simulink model "rocket"  (R2021a)
settings: Solver=VariableStepAuto  StartTime=0.0  StopTime=40  RelTol=1e-3
libraries: dspindex x5, shared3dof x3, aerolibanim x2
settings Model: Creator=scien  LastModifiedBy=scien
settings SolverCC: ZeroCrossAlgorithm=Adaptive
settings DebuggingCC: IgnoredZcDiagnostic=none

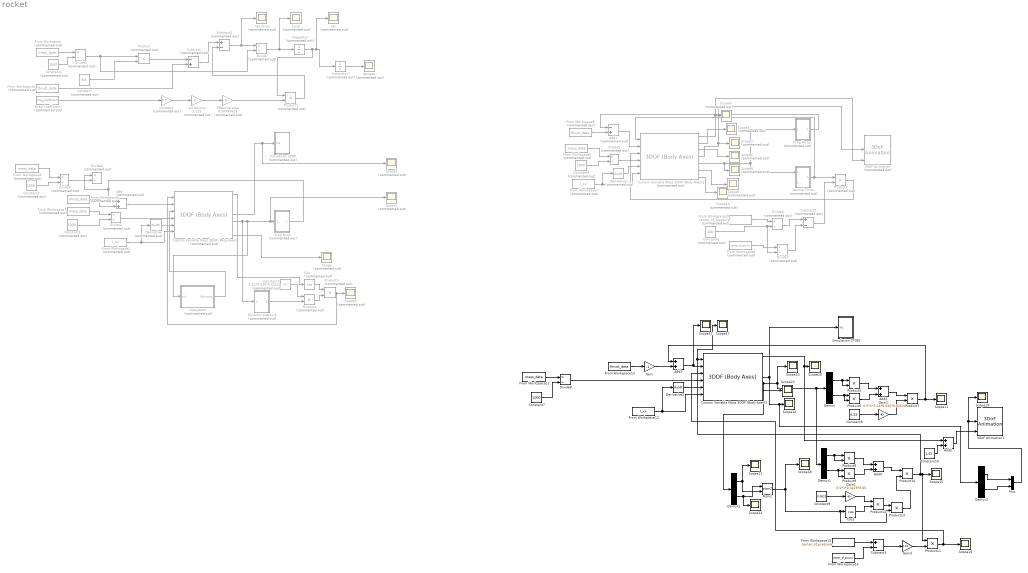
== system rocket ==
  3DoF Animation : aerolibanim/3DoF Animation  Commented=on  u1=[0 5000 -2000 2000 -5050 -3050]  u2=0.05  u3=1.0  u5=Fixed position  u6=[2000 500 -3150]  u7=10  u8=on
      settings: SourceProductBaseCode=AE
  3DoF Animation1 : aerolibanim/3DoF Animation  u1=[0 5000 -2000 2000 -5050 -3050]  u2=0.005  u3=1.0  u5=Fly alongside  u6=[0 2000 0]  u7=10  u8=on
      settings: SourceProductBaseCode=AE
  Add : Sum  Commented=on
  Add1 : Sum  Commented=on  Inputs=-+
  Add{2..5} (4 alike) : Sum
  Apogee : Scope  Commented=on
  Atan2 : Trigonometry  Operator=atan2  OutputSignalType=real
  Constant : Constant  Commented=on  Value=9.8
  Constant{1..2,4..5} (4 alike) : Constant  Commented=on  Value=1000
  Constant10 : Constant  Value=1.57
  Constant3 : Constant  Commented=on  Value=3.14*0.025*0.025/4
  Constant6 : Constant  Commented=on  Value=100
  Constant7 : Constant  Value=1000
  Constant8 : Constant  Value=6.25
  Constant9 : Constant  Value=0.0625
  Cos : Trigonometry  Commented=on  Operator=cos
  Cos1 : Trigonometry  Operator=cos
  Custom Variable Mass 3DOF (Body Axes) : shared3dof/3DOF (Body Axes)  Commented=on  units=Metric (MKS)  mtype=Custom Variable  v_ini=0  theta_ini=0  alpha_ini=0  pos_ini=[0 0]  q_ini=0  mass=1.0  mass_e=0.5  mass_f=3.0  Iyy=1.0  Iyy_e=0.5  Iyy_f=3.0  g_in=Internal  g=-9.81  vre_flag=off  abi_flag=on  aMode=0  vel_statename=''  theta_statename=''  pos_statename=''  q_statename=''  mass_statename=''
      settings: SourceProductBaseCode=AE,PW,DR,MT,UV,VE
  Custom Variable Mass 3DOF (Body Axes)1 : shared3dof/3DOF (Body Axes)  Commented=on  units=Metric (MKS)  mtype=Custom Variable  v_ini=0  theta_ini=0  alpha_ini=0  pos_ini=[0 0]  q_ini=0  mass=1.0  mass_e=0.5  mass_f=3.0  Iyy=1.0  Iyy_e=0.5  Iyy_f=3.0  g_in=Internal  g=-9.81  vre_flag=off  abi_flag=on  aMode=0  vel_statename=''  theta_statename=''  pos_statename=''  q_statename=''  mass_statename=''
      settings: SourceProductBaseCode=AE,PW,DR,MT,UV,VE
  Custom Variable Mass 3DOF (Body Axes)2 : shared3dof/3DOF (Body Axes)  units=Metric (MKS)  mtype=Custom Variable  v_ini=0  theta_ini=-0.2  alpha_ini=0  pos_ini=[0 0]  q_ini=0  mass=1.0  mass_e=0.5  mass_f=3.0  Iyy=1.0  Iyy_e=0.5  Iyy_f=3.0  g_in=Internal  g=9.81  vre_flag=off  abi_flag=on  aMode=0  vel_statename=''  theta_statename=''  pos_statename=''  q_statename=''  mass_statename=''
      settings: SourceProductBaseCode=AE,PW,DR,MT,UV,VE
  Demux{,1..3} (4 alike) : Demux  Outputs=2
  Derivative : Derivative  Commented=on
  Derivative1 : Derivative  Commented=on
  Derivative2 : Derivative
  Divide{,1..7} (8 alike) : Product  Commented=on  Inputs=*/
  Divide8 : Product  Inputs=*/
  Drag Coefficient : FromWorkspace  Commented=on  VariableName=drag_coefficient
  Drag Force : Subsystem  Commented=on
  Dynamic pressure : Subsystem  Commented=on
  Effective area : Gain  Commented=on  Gain=0.00490625
  From Workspace{,3,5..6} (4 alike) : FromWorkspace  Commented=on  VariableName=mass_data
  From Workspace1 : FromWorkspace  Commented=on  VariableName=thrust_data
  From Workspace10 : FromWorkspace  Commented=on  VariableName=center_of_pressure
  From Workspace11 : FromWorkspace  VariableName=mass_data
  From Workspace12 : FromWorkspace  VariableName=I_xx
  From Workspace13 : FromWorkspace  VariableName=thrust_data
  From Workspace14 : FromWorkspace  VariableName=center_of_gravity
  From Workspace15 : FromWorkspace  VariableName=center_of_pressure
  From Workspace2 : FromWorkspace  Commented=on  VariableName=I_xx
  From Workspace4 : FromWorkspace  Commented=on  VariableName=thrust_data
  From Workspace7 : FromWorkspace  Commented=on  VariableName=I_xx
  From Workspace8 : FromWorkspace  Commented=on  VariableName=thrust_data
  From Workspace9 : FromWorkspace  Commented=on  VariableName=center_of_gravity
  Gain : Gain  Gain=-1
  Gain1 : Gain  Gain=0.5*1*3.14*0.025*0.025/4
  Gain2 : Gain  Gain=0.5*1*0.3225*0.05
  Gain3 : Gain  Gain=0.01
  Integrator : Integrator  Commented=on
  Integrator1 : Integrator  Commented=on
  Mux : Mux  Inputs=2
  Normal Force : Subsystem  Commented=on
  Product{,1..4} (5 alike) : Product  Commented=on
  Product{5..13} (9 alike) : Product
  Scope{,1..10} (11 alike) : Scope  Commented=on
  Scope{11..23} (13 alike) : Scope
  Simulation STOP : Subsystem  Commented=on
  Simulation STOP2 : Subsystem
  Subsystem : Subsystem  Commented=on
  Subtract : Sum  Commented=on  Inputs=-+
  Subtract1 : Sum  Commented=on  Inputs=+-
  Subtract2 : Sum  Commented=on  Inputs=+-
  Subtract3 : Sum  Inputs=+-
  accel : Scope  Commented=on
  air density : Gain  Commented=on  Gain=1.225
  constant : Gain  Commented=on  Gain=0.5
  drag force : Subsystem  Commented=on
  net_force : Scope  Commented=on
  vel : Scope  Commented=on
  wires:
  Constant/1 -> Product/2
  From Workspace1/1 -> Subtract/2
  Product/1 -> Subtract/1
  Divide/1 -> accel/1, Integrator/1
  Integrator/1 -> vel/1, Integrator1/1, Product1/1
  Integrator1/1 -> Apogee/1
  Constant1/1 -> Divide1/2
  Divide1/1 -> Divide/2, Product/1
  From Workspace/1 -> Divide1/1
  Drag Coefficient/1 -> constant/1
  constant/1 -> air density/1
  air density/1 -> Effective area/1
  Effective area/1 -> Product1/2
  Subtract/1 -> Subtract1/1
  Product1/1 -> Subtract1/2
  Subtract1/1 -> net_force/1, Divide/1
  From Workspace2/1 -> Derivative/1, Custom Variable Mass 3DOF (Body Axes)/6
  Derivative/1 -> Custom Variable Mass 3DOF (Body Axes)/5
  From Workspace3/1 -> Divide2/1
  Constant4/1 -> Divide2/2
  Divide2/1 -> Custom Variable Mass 3DOF (Body Axes)/4
  From Workspace4/1 -> Add/2
  Add/1 -> Custom Variable Mass 3DOF (Body Axes)/2
  Custom Variable Mass 3DOF (Body Axes)/4 -> Simulation STOP/1(In1), Scope2/1
  drag force/1(Out2) -> Divide4/1, Add/1
  Subsystem/1(Moments) -> Custom Variable Mass 3DOF (Body Axes)/3
  From Workspace5/1 -> Divide3/1
  Constant2/1 -> Divide3/2
  Divide3/1 -> Divide4/2
  Custom Variable Mass 3DOF (Body Axes)/5 -> Dynamic pressure/1(In1), Subsystem/1(In1), Scope1/1, drag force/1(In1)
  Constant3/1 -> Product2/1
  Dynamic pressure/1(Out1) -> Product2/2
  Custom Variable Mass 3DOF (Body Axes)/1 -> Cos/1
  Cos/1 -> Product3/1
  Product2/1 -> Product3/2
  Product3/1 -> Custom Variable Mass 3DOF (Body Axes)/1, Scope3/1
  Custom Variable Mass 3DOF (Body Axes)/7 -> Scope/1
  From Workspace6/1 -> Divide5/1
  Divide5/1 -> Custom Variable Mass 3DOF (Body Axes)1/4
  Constant5/1 -> Divide5/2
  From Workspace7/1 -> Custom Variable Mass 3DOF (Body Axes)1/6, Derivative1/1
  Derivative1/1 -> Custom Variable Mass 3DOF (Body Axes)1/5
  Custom Variable Mass 3DOF (Body Axes)1/5 -> Scope8/1, Drag Force/1(In1), Normal Force/1(In1)
  From Workspace8/1 -> Add1/2
  Drag Force/1(Out3) -> Add1/1
  Add1/1 -> Custom Variable Mass 3DOF (Body Axes)1/2
  Normal Force/1(Out3) -> Custom Variable Mass 3DOF (Body Axes)1/1, Product4/1
  Divide7/1 -> Subtract2/2
  From Workspace9/1 -> Divide7/1
  Divide6/1 -> Subtract2/1
  From Workspace10/1 -> Divide6/1
  Subtract2/1 -> Product4/2
  Constant6/1 -> Divide7/2, Divide6/2
  Product4/1 -> Custom Variable Mass 3DOF (Body Axes)1/3
  Custom Variable Mass 3DOF (Body Axes)1/1 -> 3DoF Animation/3, Scope4/1
  Custom Variable Mass 3DOF (Body Axes)1/2 -> Scope5/1
  Custom Variable Mass 3DOF (Body Axes)1/3 -> Scope6/1
  Custom Variable Mass 3DOF (Body Axes)1/4 -> Scope7/1, 3DoF Animation/2
  Custom Variable Mass 3DOF (Body Axes)1/6 -> Scope9/1
  Custom Variable Mass 3DOF (Body Axes)1/7 -> Scope10/1
  From Workspace11/1 -> Divide8/1
  From Workspace12/1 -> Derivative2/1, Custom Variable Mass 3DOF (Body Axes)2/6
  Derivative2/1 -> Custom Variable Mass 3DOF (Body Axes)2/5
  Divide8/1 -> Custom Variable Mass 3DOF (Body Axes)2/4
  Constant7/1 -> Divide8/2
  From Workspace13/1 -> Gain/1
  Constant8/1 -> Gain1/1
  Custom Variable Mass 3DOF (Body Axes)2/5 -> Demux2/1, Demux1/1, Demux/1, Scope13/1
  Demux/2 -> Product6/2, Product6/1
  Product5/1 -> Add2/1
  Product6/1 -> Add2/2
  Add2/1 -> Product7/1
  Gain1/1 -> Product7/2
  Product7/1 -> Add3/1, Scope11/1
  Gain/1 -> Add3/2
  Add3/1 -> Custom Variable Mass 3DOF (Body Axes)2/2, Scope12/1
  Custom Variable Mass 3DOF (Body Axes)2/4 -> Demux3/1, Scope14/1, Simulation STOP2/1(In1)
  Add4/1 -> Product10/1
  Product9/1 -> Add4/2
  Demux1/2 -> Product9/2, Product9/1
  Product10/1 -> Scope17/1, Custom Variable Mass 3DOF (Body Axes)2/1, Product11/1, Scope15/1
  Constant9/1 -> Gain2/1
  Product8/1 -> Add4/1
  Gain2/1 -> Product12/1
  Cos1/1 -> Product12/2
  Product12/1 -> Product13/1
  Product13/1 -> Product10/2
  From Workspace15/1 -> Subtract3/1
  From Workspace14/1 -> Subtract3/2
  Subtract3/1 -> Gain3/1
  Gain3/1 -> Product11/2
  Demux/1 -> Product5/2, Product5/1
  Demux1/1 -> Product8/2, Product8/1
  Mux/1 -> Scope19/1, 3DoF Animation1/2
  Custom Variable Mass 3DOF (Body Axes)2/1 -> Add5/1, Scope20/1
  Demux2/2 -> Atan2/1, Scope22/1
  Demux2/1 -> Atan2/2, Scope21/1
  Atan2/1 -> Product13/2, Cos1/1, Scope18/1
  Product11/1 -> Custom Variable Mass 3DOF (Body Axes)2/3, Scope16/1
  Custom Variable Mass 3DOF (Body Axes)2/6 -> Scope23/1
  Demux3/2 -> Mux/2
  Demux3/1 -> Mux/1
  Constant10/1 -> Add5/2
  Add5/1 -> 3DoF Animation1/3

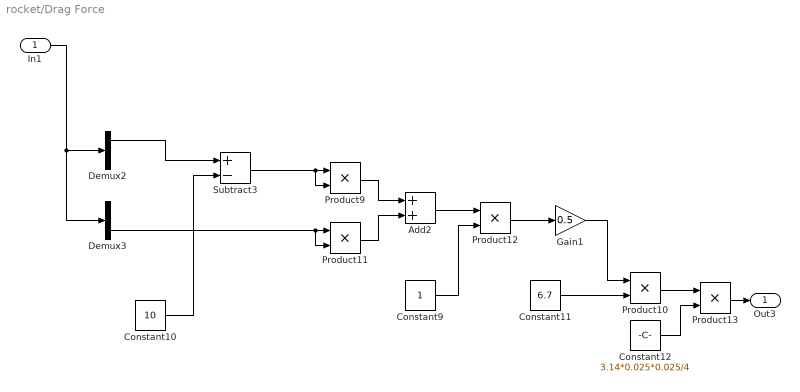
== system rocket/Drag Force ==
  In1 : Inport
  Add2 : Sum
  Constant10 : Constant  Value=10
  Constant11 : Constant  Value=6.7
  Constant12 : Constant  Value=3.14*0.025*0.025/4
  Constant9 : Constant
  Demux2 : Demux  Outputs=2
  Demux3 : Demux  Outputs=2
  Gain1 : Gain  Gain=0.5
  Product{9..13} (5 alike) : Product
  Subtract3 : Sum  Inputs=+-
  Out3 : Outport
  wires:
  Demux2/1 -> Subtract3/1
  Product11/1 -> Add2/2
  In1/1 -> Demux3/1, Demux2/1
  Constant10/1 -> Subtract3/2
  Subtract3/1 -> Product9/2, Product9/1
  Add2/1 -> Product12/1
  Gain1/1 -> Product10/1
  Product9/1 -> Add2/1
  Demux3/2 -> Product11/2, Product11/1
  Constant9/1 -> Product12/2
  Product10/1 -> Product13/1
  Product12/1 -> Gain1/1
  Constant11/1 -> Product10/2
  Constant12/1 -> Product13/2
  Product13/1 -> Out3/1

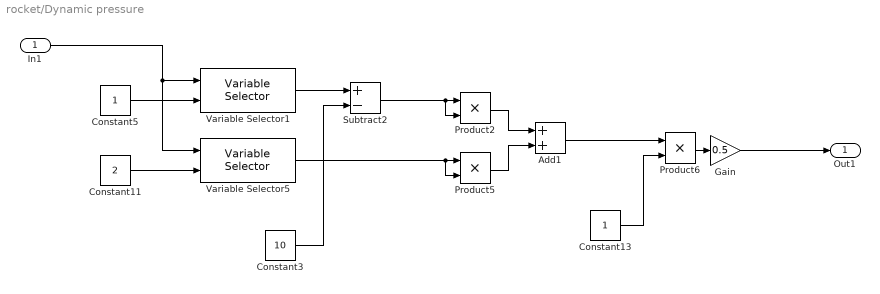
== system rocket/Dynamic pressure ==
  In1 : Inport
  Add1 : Sum
  Constant11 : Constant  Value=2
  Constant13 : Constant
  Constant3 : Constant  Value=10
  Constant5 : Constant
  Gain : Gain  Gain=0.5
  Product2 : Product
  Product5 : Product
  Product6 : Product
  Subtract2 : Sum  Inputs=+-
  Variable Selector1 : dspindex/Variable Selector  NumInputs=1  rowsOrCols=Rows  IdxMode=Variable  Elements=[1 3]  ZerOneIdxMode=One-based  errmode=Clip Index  FillMode=on  FillValues=0
  Variable Selector5 : dspindex/Variable Selector  NumInputs=1  rowsOrCols=Rows  IdxMode=Variable  Elements=[1 3]  ZerOneIdxMode=One-based  errmode=Clip Index  FillMode=on  FillValues=0
  Out1 : Outport
  wires:
  Constant5/1 -> Variable Selector1/2
  Product5/1 -> Add1/2
  Variable Selector1/1 -> Subtract2/1
  Variable Selector5/1 -> Product5/2, Product5/1
  Subtract2/1 -> Product2/2, Product2/1
  In1/1 -> Variable Selector5/1, Variable Selector1/1
  Constant3/1 -> Subtract2/2
  Product2/1 -> Add1/1
  Constant13/1 -> Product6/2
  Product6/1 -> Gain/1
  Constant11/1 -> Variable Selector5/2
  Add1/1 -> Product6/1
  Gain/1 -> Out1/1

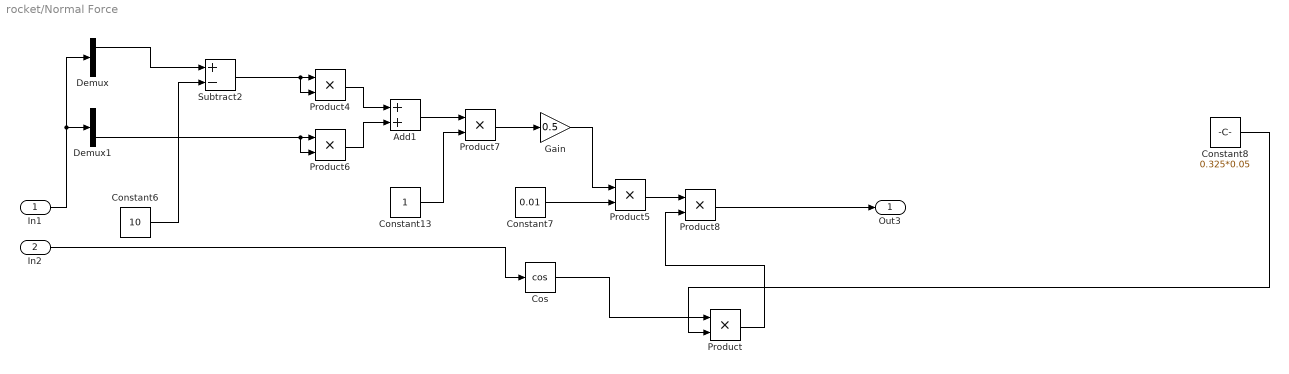
== system rocket/Normal Force ==
  In1 : Inport
  In2 : Inport  Port=2
  Add1 : Sum
  Constant13 : Constant
  Constant6 : Constant  Value=10
  Constant7 : Constant  Value=0.01
  Constant8 : Constant  Value=0.325*0.05
  Cos : Trigonometry  Operator=cos
  Demux : Demux  Outputs=2
  Demux1 : Demux  Outputs=2
  Gain : Gain  Gain=0.5
  Product{,4..8} (6 alike) : Product
  Subtract2 : Sum  Inputs=+-
  Out3 : Outport
  wires:
  In1/1 -> Demux/1, Demux1/1
  Constant6/1 -> Subtract2/2
  Add1/1 -> Product7/1
  Constant7/1 -> Product5/2
  Constant13/1 -> Product7/2
  Product5/1 -> Product8/1
  Product7/1 -> Gain/1
  Demux1/2 -> Product6/2, Product6/1
  Product4/1 -> Add1/1
  Subtract2/1 -> Product4/2, Product4/1
  Gain/1 -> Product5/1
  Product6/1 -> Add1/2
  Demux/1 -> Subtract2/1
  Product8/1 -> Out3/1
  Cos/1 -> Product/1
  In2/1 -> Cos/1
  Constant8/1 -> Product/2
  Product/1 -> Product8/2

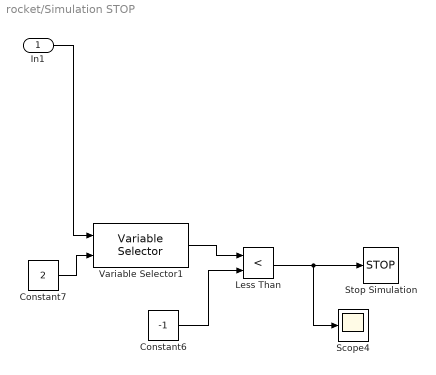
== system rocket/Simulation STOP ==
  In1 : Inport
  Constant6 : Constant  Value=-1
  Constant7 : Constant  Value=2
  Less Than : RelationalOperator  Operator=<  OutDataTypeStr=boolean  RndMeth=Simplest
  Scope4 : Scope
  Stop Simulation : Stop
  Variable Selector1 : dspindex/Variable Selector  NumInputs=1  rowsOrCols=Rows  IdxMode=Variable  Elements=[1 3]  ZerOneIdxMode=One-based  errmode=Clip Index  FillMode=on  FillValues=0
  wires:
  Less Than/1 -> Scope4/1, Stop Simulation/1
  In1/1 -> Variable Selector1/1
  Variable Selector1/1 -> Less Than/1
  Constant6/1 -> Less Than/2
  Constant7/1 -> Variable Selector1/2

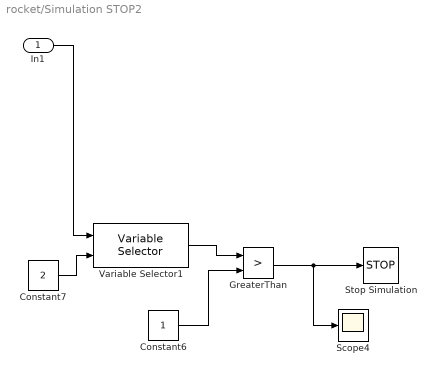
== system rocket/Simulation STOP2 ==
  In1 : Inport
  Constant6 : Constant
  Constant7 : Constant  Value=2
  GreaterThan : RelationalOperator  Operator=>  OutDataTypeStr=boolean  RndMeth=Simplest
  Scope4 : Scope
  Stop Simulation : Stop
  Variable Selector1 : dspindex/Variable Selector  NumInputs=1  rowsOrCols=Rows  IdxMode=Variable  Elements=[1 3]  ZerOneIdxMode=One-based  errmode=Clip Index  FillMode=on  FillValues=0
  wires:
  Constant7/1 -> Variable Selector1/2
  Constant6/1 -> GreaterThan/2
  Variable Selector1/1 -> GreaterThan/1
  In1/1 -> Variable Selector1/1
  GreaterThan/1 -> Stop Simulation/1, Scope4/1

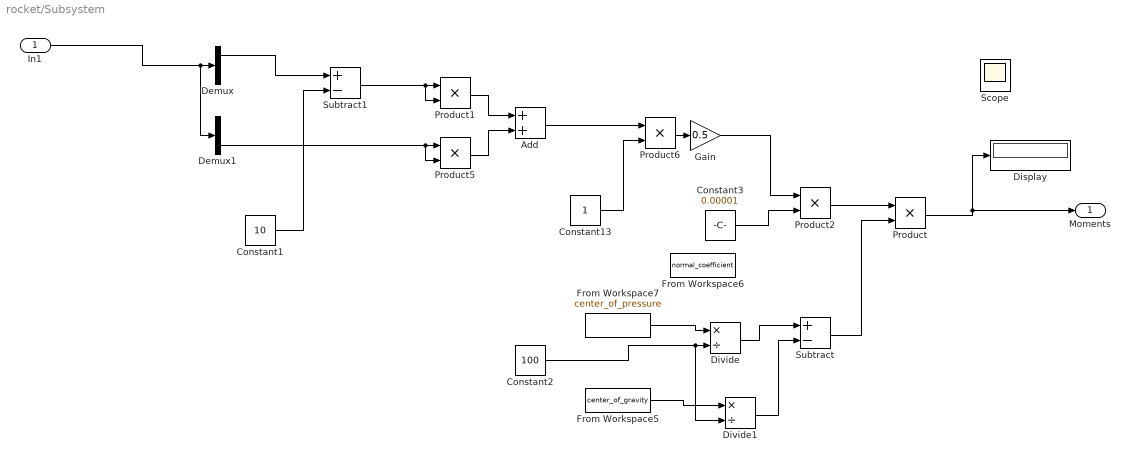
== system rocket/Subsystem ==
  In1 : Inport
  Add : Sum
  Constant1 : Constant  Value=10
  Constant13 : Constant
  Constant2 : Constant  Value=100
  Constant3 : Constant  Value=0.00001
  Demux : Demux  Outputs=2
  Demux1 : Demux  Outputs=2
  Display : Display
  Divide : Product  Inputs=*/
  Divide1 : Product  Inputs=*/
  From Workspace5 : FromWorkspace  VariableName=center_of_gravity
  From Workspace6 : FromWorkspace  VariableName=normal_coefficient
  From Workspace7 : FromWorkspace  VariableName=center_of_pressure
  Gain : Gain  Gain=0.5
  Product{,1..2,5..6} (5 alike) : Product
  Scope : Scope
  Subtract : Sum  Inputs=+-
  Subtract1 : Sum  Inputs=+-
  Moments : Outport
  wires:
  In1/1 -> Demux1/1, Demux/1
  Gain/1 -> Product2/1
  Constant13/1 -> Product6/2
  Subtract/1 -> Product/2
  Product2/1 -> Product/1
  Demux/1 -> Subtract1/1
  Constant1/1 -> Subtract1/2
  Subtract1/1 -> Product1/2, Product1/1
  Demux1/2 -> Product5/2, Product5/1
  Product1/1 -> Add/1
  Product5/1 -> Add/2
  Add/1 -> Product6/1
  Product6/1 -> Gain/1
  Product/1 -> Moments/1, Display/1
  From Workspace7/1 -> Divide/1
  From Workspace5/1 -> Divide1/1
  Constant2/1 -> Divide1/2, Divide/2
  Divide1/1 -> Subtract/2
  Divide/1 -> Subtract/1
  Constant3/1 -> Product2/2

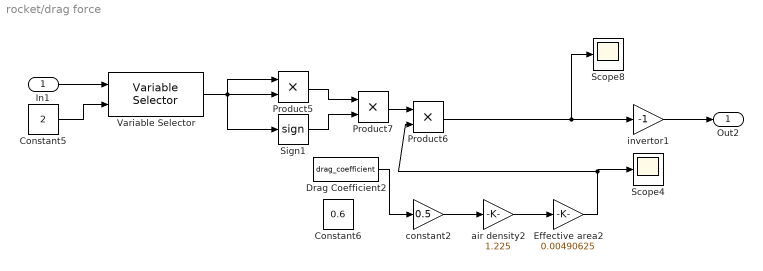
== system rocket/drag force ==
  In1 : Inport
  Constant5 : Constant  Value=2
  Constant6 : Constant  Value=0.6
  Drag Coefficient2 : FromWorkspace  VariableName=drag_coefficient
  Effective area2 : Gain  Gain=0.00490625
  Product5 : Product
  Product6 : Product
  Product7 : Product
  Scope4 : Scope
  Scope8 : Scope
  Sign1 : Signum
  Variable Selector : dspindex/Variable Selector  NumInputs=1  rowsOrCols=Rows  IdxMode=Variable  Elements=[1 3]  ZerOneIdxMode=One-based  errmode=Clip Index  FillMode=on  FillValues=0
  air density2 : Gain  Gain=1.225
  constant2 : Gain  Gain=0.5
  invertor1 : Gain  Gain=-1
  Out2 : Outport
  wires:
  Constant5/1 -> Variable Selector/2
  air density2/1 -> Effective area2/1
  Product7/1 -> Product6/1
  Variable Selector/1 -> Product5/1, Sign1/1, Product5/2
  invertor1/1 -> Out2/1
  Product6/1 -> invertor1/1, Scope8/1
  constant2/1 -> air density2/1
  Effective area2/1 -> Scope4/1, Product6/2
  Sign1/1 -> Product7/2
  Product5/1 -> Product7/1
  In1/1 -> Variable Selector/1
  Drag Coefficient2/1 -> constant2/1
